simulink model "ACC_Scenario_006_cs"  (R2014b)
settings: Solver=ode5  SolverMode=SingleTasking  StartTime=0.0  StopTime=inf  FixedStep=1/100  RelTol=1e-3
PreLoadFcn:
  | mbxruntime.callbacks.PreLoadFcn(bdroot);
  | check_NUTS_defined;
  | 
  | assignin('base',['model_closed_' bdroot],false);addpath('../includes_ACC');
PostLoadFcn:
  | mbxruntime.callbacks.PostLoadFcn(bdroot);
InitFcn:
  | mbxruntime.callbacks.InitFcn(bdroot);
StartFcn:
  | mbxruntime.callbacks.StartFcn(bdroot);
StopFcn:
  | mbxruntime.callbacks.StopFcn(bdroot);
model workspace: external: MAT-File .\ACC_Scenario_006_cs_hws.mat (data not in the file)
undefined symbols (not defined in the file or in its folder): mbxruntime, OrientationPitch, OrientationRoll, PositionX, PositionY, PositionZ, tabledata, warningInitialVelocity, x0
undefined symbols (not defined in the file): ACC_Scenario_006_cs_061450488d6753c4, ACC_Scenario_006_cs_13896134c615b72a, ACC_Scenario_006_cs_18eaf2a52f2ef75d, ACC_Scenario_006_cs_59e375456829d2f0, ACC_Scenario_006_cs_8a2109b915871f11, ACC_Scenario_006_cs_a4f79cab717c06e2, ACC_Scenario_006_cs_Audi_A8_1_Dynamics_Simple_initialPitch, ACC_Scenario_006_cs_Audi_A8_1_Dynamics_Simple_initialRoll, ACC_Scenario_006_cs_Audi_A8_1_Dynamics_Simple_initialX, ACC_Scenario_006_cs_Audi_A8_1_Dynamics_Simple_initialY, ACC_Scenario_006_cs_Audi_A8_1_Dynamics_Simple_initialYaw, ACC_Scenario_006_cs_Audi_A8_1_Dynamics_Simple_initialZ, ACC_Scenario_006_cs_BMW_X5_1_Path_pathUniqueID, ACC_Scenario_006_cs_BMW_X5_1_SpeedProfile_speedProfileUniqueID, ACC_Scenario_006_cs_e4633c18fd34a832, ACC_Scenario_006_cs_f83c81dc10cd364a, ACC_Scenario_006_cs_Fiat_Bravo_1_Path_pathUniqueID, ACC_Scenario_006_cs_Ford_Fiesta_1_Path_pathUniqueID, ACC_Scenario_006_cs_Honda_Pan_European_1_Path_pathUniqueID, ACC_Scenario_006_cs_Mazda_RX8_1_Path_pathUniqueID, ACC_Scenario_006_cs_Sphere_1_Dynamics_Empty_STATE_Sphere_1_x0, ACC_Scenario_006_cs_Sphere_1_Dynamics_Empty_STATE_Sphere_1_y0, ACC_Scenario_006_cs_Sphere_1_Dynamics_Empty_STATE_Sphere_1_Yaw0, ACC_Scenario_006_cs_Sphere_1_Dynamics_Empty_STATE_Sphere_1_z0, ACC_Scenario_006_cs_Toyota_Yaris_1_Path_pathUniqueID, SteeringColumn, SteeringWheel, Wheel0, Wheel0_Suspension, Wheel1, Wheel1_Suspension, WheelL0, WheelL1, WheelR0, WheelR1
libraries: simulink_extras x60, simulink x21, PreScanSimulinkLibrary x5, PreScanUsefulBlocks x2
(part 6 of 24)

== system ACC_Scenario_006_cs/HighwayOverhang_12 ==
  note: Resources
      |
      | 1: InformationSign\MatrixSign_GreenArrow.png: MatrixSign GreenArrow
      | 2: InformationSign\sign1.jpg: sign1
      | 3: InformationSign\sign2.jpg: sign2
      | 4: InformationSign\sign3.jpg: sign3
      | 5: InformationSign\sign10.png: sign10
      | 7: InformationSign\SEARCH_Logo.png: SEARCH Logo
      | 8: InformationSign\sharp_edges.jpg: sharp edges
      | 9: InformationSign\road_surprises.jpg: road surprises
      | 10: InformationSign\sign5.JPG: sign5
      | 11: InformationSign\tacos.jpg: tacos
      | 12: InformationSign\dont_even_think.jpg: dont even think
      | 13: InformationSign\cthulhuwarn.jpg: cthulhuwarn
      | 14: InformationSign\sign7.JPG: sign7
      | 15: InformationSign\sign32.jpg: sign32
      | 16: InformationSign\NoParking.jpg: NoParking
      | 17: InformationSign\TheFuture.jpg: TheFuture
      | 18: InformationSign\sign4.jpg: sign4
      | 19: InformationSign\sign31.jpg: sign31
      | 20: InformationSign\Empty.jpeg: Empty
  Ground_{1..4} (4 alike) : Ground
  VISUMatrixSignLights_Mux : Subsystem  Tag=mux/VisuMatrixSignLights  mask(PreScan User Interface: VisuMatrixSignLights){}
      mask help:
      | The VisuMatrixSignLights block provides a way to switch the lights on the matrix sign board on or off
      |
      | For more information, please click Help.
      mask Help: eval('openHelp(732)')
  VISUMatrixSign_Mux : Subsystem  Tag=mux/MatrixSign_v2  mask(PreScan User Interface: VisuMatrixSign){}
      mask help:
      | The VisuMatrixSign block provides a way to adapt the texture of the plates connected to an overhang, based on Resource IDs of the texture files.
      |
      | For more information, please click Help.
      settings: DeleteFcn=PreScanBlockDeleteFcn;
      mask Help: eval('openHelp(733)')
  VISUMatrixSign_HighwayOverhang_12 : Outport  Tag=outport/VisuMatrixSign  SampleTime=1/100
  VISUMatrixSignLights_HighwayOverhang_12 : Outport  Tag=outport/VisuMatrixSignLights  Port=2  SampleTime=1/100
  wires:
  VISUMatrixSign_Mux/1(MatrixSigns) -> VISUMatrixSign_HighwayOverhang_12/1
  VISUMatrixSignLights_Mux/1(VISUMatrixSignLights_HighwayOverhang_12) -> VISUMatrixSignLights_HighwayOverhang_12/1
  Ground_1/1 -> VISUMatrixSignLights_Mux/1(MatrixSign_5)
  Ground_2/1 -> VISUMatrixSignLights_Mux/2(MatrixSign_6)
  Ground_3/1 -> VISUMatrixSign_Mux/1(MatrixSign_5)
  Ground_4/1 -> VISUMatrixSign_Mux/2(MatrixSign_6)

== system ACC_Scenario_006_cs/HighwayOverhang_2 ==
  note: Resources
      |
      | 1: InformationSign\MatrixSign_GreenArrow.png: MatrixSign GreenArrow
      | 2: InformationSign\sign1.jpg: sign1
      | 3: InformationSign\sign2.jpg: sign2
      | 4: InformationSign\sign3.jpg: sign3
      | 5: InformationSign\sign10.png: sign10
      | 7: InformationSign\SEARCH_Logo.png: SEARCH Logo
      | 8: InformationSign\sharp_edges.jpg: sharp edges
      | 9: InformationSign\road_surprises.jpg: road surprises
      | 10: InformationSign\sign5.JPG: sign5
      | 11: InformationSign\tacos.jpg: tacos
      | 12: InformationSign\dont_even_think.jpg: dont even think
      | 13: InformationSign\cthulhuwarn.jpg: cthulhuwarn
      | 14: InformationSign\sign7.JPG: sign7
      | 15: InformationSign\sign32.jpg: sign32
      | 16: InformationSign\NoParking.jpg: NoParking
      | 17: InformationSign\TheFuture.jpg: TheFuture
      | 18: InformationSign\sign4.jpg: sign4
      | 19: InformationSign\sign31.jpg: sign31
      | 20: InformationSign\Empty.jpeg: Empty
  Ground_{1..4} (4 alike) : Ground
  VISUMatrixSignLights_Mux : Subsystem  Tag=mux/VisuMatrixSignLights  mask(PreScan User Interface: VisuMatrixSignLights){}
      mask help:
      | The VisuMatrixSignLights block provides a way to switch the lights on the matrix sign board on or off
      |
      | For more information, please click Help.
      mask Help: eval('openHelp(732)')
  VISUMatrixSign_Mux : Subsystem  Tag=mux/MatrixSign_v2  mask(PreScan User Interface: VisuMatrixSign){}
      mask help:
      | The VisuMatrixSign block provides a way to adapt the texture of the plates connected to an overhang, based on Resource IDs of the texture files.
      |
      | For more information, please click Help.
      settings: DeleteFcn=PreScanBlockDeleteFcn;
      mask Help: eval('openHelp(733)')
  VISUMatrixSign_HighwayOverhang_2 : Outport  Tag=outport/VisuMatrixSign  SampleTime=1/100
  VISUMatrixSignLights_HighwayOverhang_2 : Outport  Tag=outport/VisuMatrixSignLights  Port=2  SampleTime=1/100
  wires:
  VISUMatrixSign_Mux/1(MatrixSigns) -> VISUMatrixSign_HighwayOverhang_2/1
  VISUMatrixSignLights_Mux/1(VISUMatrixSignLights_HighwayOverhang_2) -> VISUMatrixSignLights_HighwayOverhang_2/1
  Ground_1/1 -> VISUMatrixSignLights_Mux/1(MatrixSign_3)
  Ground_2/1 -> VISUMatrixSignLights_Mux/2(MatrixSign_4)
  Ground_3/1 -> VISUMatrixSign_Mux/1(MatrixSign_3)
  Ground_4/1 -> VISUMatrixSign_Mux/2(MatrixSign_4)

== system ACC_Scenario_006_cs/HighwayOverhang_3 ==
  note: Resources
      |
      | 1: InformationSign\MatrixSign_GreenArrow.png: MatrixSign GreenArrow
      | 2: InformationSign\sign1.jpg: sign1
      | 3: InformationSign\sign2.jpg: sign2
      | 4: InformationSign\sign3.jpg: sign3
      | 5: InformationSign\sign10.png: sign10
      | 7: InformationSign\SEARCH_Logo.png: SEARCH Logo
      | 8: InformationSign\sharp_edges.jpg: sharp edges
      | 9: InformationSign\road_surprises.jpg: road surprises
      | 10: InformationSign\sign5.JPG: sign5
      | 11: InformationSign\tacos.jpg: tacos
      | 12: InformationSign\dont_even_think.jpg: dont even think
      | 13: InformationSign\cthulhuwarn.jpg: cthulhuwarn
      | 14: InformationSign\sign7.JPG: sign7
      | 15: InformationSign\sign32.jpg: sign32
      | 16: InformationSign\NoParking.jpg: NoParking
      | 17: InformationSign\TheFuture.jpg: TheFuture
      | 18: InformationSign\sign4.jpg: sign4
      | 19: InformationSign\sign31.jpg: sign31
      | 20: InformationSign\Empty.jpeg: Empty
  Ground_1 : Ground
  Ground_2 : Ground
  VISUMatrixSign_Mux : Subsystem  Tag=mux/MatrixSign_v2  mask(PreScan User Interface: VisuMatrixSign){}
      mask help:
      | The VisuMatrixSign block provides a way to adapt the texture of the plates connected to an overhang, based on Resource IDs of the texture files.
      |
      | For more information, please click Help.
      settings: DeleteFcn=PreScanBlockDeleteFcn;
      mask Help: eval('openHelp(733)')
  VISUMatrixSign_HighwayOverhang_3 : Outport  Tag=outport/VisuMatrixSign  SampleTime=1/100
  wires:
  VISUMatrixSign_Mux/1(MatrixSigns) -> VISUMatrixSign_HighwayOverhang_3/1
  Ground_1/1 -> VISUMatrixSign_Mux/1(InformationPlate_1)
  Ground_2/1 -> VISUMatrixSign_Mux/2(InformationPlate_2)

== system ACC_Scenario_006_cs/HighwayOverhang_4 ==
  note: Resources
      |
      | 1: InformationSign\MatrixSign_GreenArrow.png: MatrixSign GreenArrow
      | 2: InformationSign\sign1.jpg: sign1
      | 3: InformationSign\sign2.jpg: sign2
      | 4: InformationSign\sign3.jpg: sign3
      | 5: InformationSign\sign10.png: sign10
      | 7: InformationSign\SEARCH_Logo.png: SEARCH Logo
      | 8: InformationSign\sharp_edges.jpg: sharp edges
      | 9: InformationSign\road_surprises.jpg: road surprises
      | 10: InformationSign\sign5.JPG: sign5
      | 11: InformationSign\tacos.jpg: tacos
      | 12: InformationSign\dont_even_think.jpg: dont even think
      | 13: InformationSign\cthulhuwarn.jpg: cthulhuwarn
      | 14: InformationSign\sign7.JPG: sign7
      | 15: InformationSign\sign32.jpg: sign32
      | 16: InformationSign\NoParking.jpg: NoParking
      | 17: InformationSign\TheFuture.jpg: TheFuture
      | 18: InformationSign\sign4.jpg: sign4
      | 19: InformationSign\sign31.jpg: sign31
      | 20: InformationSign\Empty.jpeg: Empty
  Ground_1 : Ground
  Ground_2 : Ground
  VISUMatrixSign_Mux : Subsystem  Tag=mux/MatrixSign_v2  mask(PreScan User Interface: VisuMatrixSign){}
      mask help:
      | The VisuMatrixSign block provides a way to adapt the texture of the plates connected to an overhang, based on Resource IDs of the texture files.
      |
      | For more information, please click Help.
      settings: DeleteFcn=PreScanBlockDeleteFcn;
      mask Help: eval('openHelp(733)')
  VISUMatrixSign_HighwayOverhang_4 : Outport  Tag=outport/VisuMatrixSign  SampleTime=1/100
  wires:
  VISUMatrixSign_Mux/1(MatrixSigns) -> VISUMatrixSign_HighwayOverhang_4/1
  Ground_1/1 -> VISUMatrixSign_Mux/1(InformationPlate_3)
  Ground_2/1 -> VISUMatrixSign_Mux/2(InformationPlate_4)

== system ACC_Scenario_006_cs/HighwayOverhang_5 ==
  note: Resources
      |
      | 1: InformationSign\MatrixSign_GreenArrow.png: MatrixSign GreenArrow
      | 2: InformationSign\sign1.jpg: sign1
      | 3: InformationSign\sign2.jpg: sign2
      | 4: InformationSign\sign3.jpg: sign3
      | 5: InformationSign\sign10.png: sign10
      | 7: InformationSign\SEARCH_Logo.png: SEARCH Logo
      | 8: InformationSign\sharp_edges.jpg: sharp edges
      | 9: InformationSign\road_surprises.jpg: road surprises
      | 10: InformationSign\sign5.JPG: sign5
      | 11: InformationSign\tacos.jpg: tacos
      | 12: InformationSign\dont_even_think.jpg: dont even think
      | 13: InformationSign\cthulhuwarn.jpg: cthulhuwarn
      | 14: InformationSign\sign7.JPG: sign7
      | 15: InformationSign\sign32.jpg: sign32
      | 16: InformationSign\NoParking.jpg: NoParking
      | 17: InformationSign\TheFuture.jpg: TheFuture
      | 18: InformationSign\sign4.jpg: sign4
      | 19: InformationSign\sign31.jpg: sign31
      | 20: InformationSign\Empty.jpeg: Empty
  Ground_1 : Ground
  Ground_2 : Ground
  VISUMatrixSign_Mux : Subsystem  Tag=mux/MatrixSign_v2  mask(PreScan User Interface: VisuMatrixSign){}
      mask help:
      | The VisuMatrixSign block provides a way to adapt the texture of the plates connected to an overhang, based on Resource IDs of the texture files.
      |
      | For more information, please click Help.
      settings: DeleteFcn=PreScanBlockDeleteFcn;
      mask Help: eval('openHelp(733)')
  VISUMatrixSign_HighwayOverhang_5 : Outport  Tag=outport/VisuMatrixSign  SampleTime=1/100
  wires:
  VISUMatrixSign_Mux/1(MatrixSigns) -> VISUMatrixSign_HighwayOverhang_5/1
  Ground_1/1 -> VISUMatrixSign_Mux/1(InformationPlate_5)
  Ground_2/1 -> VISUMatrixSign_Mux/2(InformationPlate_6)

== system ACC_Scenario_006_cs/HighwayOverhang_6 ==
  note: Resources
      |
      | 1: InformationSign\MatrixSign_GreenArrow.png: MatrixSign GreenArrow
      | 2: InformationSign\sign1.jpg: sign1
      | 3: InformationSign\sign2.jpg: sign2
      | 4: InformationSign\sign3.jpg: sign3
      | 5: InformationSign\sign10.png: sign10
      | 7: InformationSign\SEARCH_Logo.png: SEARCH Logo
      | 8: InformationSign\sharp_edges.jpg: sharp edges
      | 9: InformationSign\road_surprises.jpg: road surprises
      | 10: InformationSign\sign5.JPG: sign5
      | 11: InformationSign\tacos.jpg: tacos
      | 12: InformationSign\dont_even_think.jpg: dont even think
      | 13: InformationSign\cthulhuwarn.jpg: cthulhuwarn
      | 14: InformationSign\sign7.JPG: sign7
      | 15: InformationSign\sign32.jpg: sign32
      | 16: InformationSign\NoParking.jpg: NoParking
      | 17: InformationSign\TheFuture.jpg: TheFuture
      | 18: InformationSign\sign4.jpg: sign4
      | 19: InformationSign\sign31.jpg: sign31
      | 20: InformationSign\Empty.jpeg: Empty
  Ground_1 : Ground
  Ground_2 : Ground
  VISUMatrixSign_Mux : Subsystem  Tag=mux/MatrixSign_v2  mask(PreScan User Interface: VisuMatrixSign){}
      mask help:
      | The VisuMatrixSign block provides a way to adapt the texture of the plates connected to an overhang, based on Resource IDs of the texture files.
      |
      | For more information, please click Help.
      settings: DeleteFcn=PreScanBlockDeleteFcn;
      mask Help: eval('openHelp(733)')
  VISUMatrixSign_HighwayOverhang_6 : Outport  Tag=outport/VisuMatrixSign  SampleTime=1/100
  wires:
  VISUMatrixSign_Mux/1(MatrixSigns) -> VISUMatrixSign_HighwayOverhang_6/1
  Ground_1/1 -> VISUMatrixSign_Mux/1(InformationPlate_7)
  Ground_2/1 -> VISUMatrixSign_Mux/2(InformationPlate_8)

== system ACC_Scenario_006_cs/HighwayOverhang_7 ==
  note: Resources
      |
      | 1: InformationSign\MatrixSign_GreenArrow.png: MatrixSign GreenArrow
      | 2: InformationSign\sign1.jpg: sign1
      | 3: InformationSign\sign2.jpg: sign2
      | 4: InformationSign\sign3.jpg: sign3
      | 5: InformationSign\sign10.png: sign10
      | 7: InformationSign\SEARCH_Logo.png: SEARCH Logo
      | 8: InformationSign\sharp_edges.jpg: sharp edges
      | 9: InformationSign\road_surprises.jpg: road surprises
      | 10: InformationSign\sign5.JPG: sign5
      | 11: InformationSign\tacos.jpg: tacos
      | 12: InformationSign\dont_even_think.jpg: dont even think
      | 13: InformationSign\cthulhuwarn.jpg: cthulhuwarn
      | 14: InformationSign\sign7.JPG: sign7
      | 15: InformationSign\sign32.jpg: sign32
      | 16: InformationSign\NoParking.jpg: NoParking
      | 17: InformationSign\TheFuture.jpg: TheFuture
      | 18: InformationSign\sign4.jpg: sign4
      | 19: InformationSign\sign31.jpg: sign31
      | 20: InformationSign\Empty.jpeg: Empty
  Ground_1 : Ground
  Ground_2 : Ground
  VISUMatrixSign_Mux : Subsystem  Tag=mux/MatrixSign_v2  mask(PreScan User Interface: VisuMatrixSign){}
      mask help:
      | The VisuMatrixSign block provides a way to adapt the texture of the plates connected to an overhang, based on Resource IDs of the texture files.
      |
      | For more information, please click Help.
      settings: DeleteFcn=PreScanBlockDeleteFcn;
      mask Help: eval('openHelp(733)')
  VISUMatrixSign_HighwayOverhang_7 : Outport  Tag=outport/VisuMatrixSign  SampleTime=1/100
  wires:
  VISUMatrixSign_Mux/1(MatrixSigns) -> VISUMatrixSign_HighwayOverhang_7/1
  Ground_1/1 -> VISUMatrixSign_Mux/1(InformationPlate_9)
  Ground_2/1 -> VISUMatrixSign_Mux/2(InformationPlate_10)

== system ACC_Scenario_006_cs/HighwayOverhang_8 ==
  note: Resources
      |
      | 1: InformationSign\MatrixSign_GreenArrow.png: MatrixSign GreenArrow
      | 2: InformationSign\sign1.jpg: sign1
      | 3: InformationSign\sign2.jpg: sign2
      | 4: InformationSign\sign3.jpg: sign3
      | 5: InformationSign\sign10.png: sign10
      | 7: InformationSign\SEARCH_Logo.png: SEARCH Logo
      | 8: InformationSign\sharp_edges.jpg: sharp edges
      | 9: InformationSign\road_surprises.jpg: road surprises
      | 10: InformationSign\sign5.JPG: sign5
      | 11: InformationSign\tacos.jpg: tacos
      | 12: InformationSign\dont_even_think.jpg: dont even think
      | 13: InformationSign\cthulhuwarn.jpg: cthulhuwarn
      | 14: InformationSign\sign7.JPG: sign7
      | 15: InformationSign\sign32.jpg: sign32
      | 16: InformationSign\NoParking.jpg: NoParking
      | 17: InformationSign\TheFuture.jpg: TheFuture
      | 18: InformationSign\sign4.jpg: sign4
      | 19: InformationSign\sign31.jpg: sign31
      | 20: InformationSign\Empty.jpeg: Empty
  Ground_1 : Ground
  Ground_2 : Ground
  VISUMatrixSign_Mux : Subsystem  Tag=mux/MatrixSign_v2  mask(PreScan User Interface: VisuMatrixSign){}
      mask help:
      | The VisuMatrixSign block provides a way to adapt the texture of the plates connected to an overhang, based on Resource IDs of the texture files.
      |
      | For more information, please click Help.
      settings: DeleteFcn=PreScanBlockDeleteFcn;
      mask Help: eval('openHelp(733)')
  VISUMatrixSign_HighwayOverhang_8 : Outport  Tag=outport/VisuMatrixSign  SampleTime=1/100
  wires:
  VISUMatrixSign_Mux/1(MatrixSigns) -> VISUMatrixSign_HighwayOverhang_8/1
  Ground_1/1 -> VISUMatrixSign_Mux/1(InformationPlate_11)
  Ground_2/1 -> VISUMatrixSign_Mux/2(InformationPlate_12)

== system ACC_Scenario_006_cs/HighwayOverhang_9 ==
  note: Resources
      |
      | 1: InformationSign\MatrixSign_GreenArrow.png: MatrixSign GreenArrow
      | 2: InformationSign\sign1.jpg: sign1
      | 3: InformationSign\sign2.jpg: sign2
      | 4: InformationSign\sign3.jpg: sign3
      | 5: InformationSign\sign10.png: sign10
      | 7: InformationSign\SEARCH_Logo.png: SEARCH Logo
      | 8: InformationSign\sharp_edges.jpg: sharp edges
      | 9: InformationSign\road_surprises.jpg: road surprises
      | 10: InformationSign\sign5.JPG: sign5
      | 11: InformationSign\tacos.jpg: tacos
      | 12: InformationSign\dont_even_think.jpg: dont even think
      | 13: InformationSign\cthulhuwarn.jpg: cthulhuwarn
      | 14: InformationSign\sign7.JPG: sign7
      | 15: InformationSign\sign32.jpg: sign32
      | 16: InformationSign\NoParking.jpg: NoParking
      | 17: InformationSign\TheFuture.jpg: TheFuture
      | 18: InformationSign\sign4.jpg: sign4
      | 19: InformationSign\sign31.jpg: sign31
      | 20: InformationSign\Empty.jpeg: Empty
  Ground_1 : Ground
  Ground_2 : Ground
  VISUMatrixSign_Mux : Subsystem  Tag=mux/MatrixSign_v2  mask(PreScan User Interface: VisuMatrixSign){}
      mask help:
      | The VisuMatrixSign block provides a way to adapt the texture of the plates connected to an overhang, based on Resource IDs of the texture files.
      |
      | For more information, please click Help.
      settings: DeleteFcn=PreScanBlockDeleteFcn;
      mask Help: eval('openHelp(733)')
  VISUMatrixSign_HighwayOverhang_9 : Outport  Tag=outport/VisuMatrixSign  SampleTime=1/100
  wires:
  VISUMatrixSign_Mux/1(MatrixSigns) -> VISUMatrixSign_HighwayOverhang_9/1
  Ground_1/1 -> VISUMatrixSign_Mux/1(InformationPlate_13)
  Ground_2/1 -> VISUMatrixSign_Mux/2(InformationPlate_14)

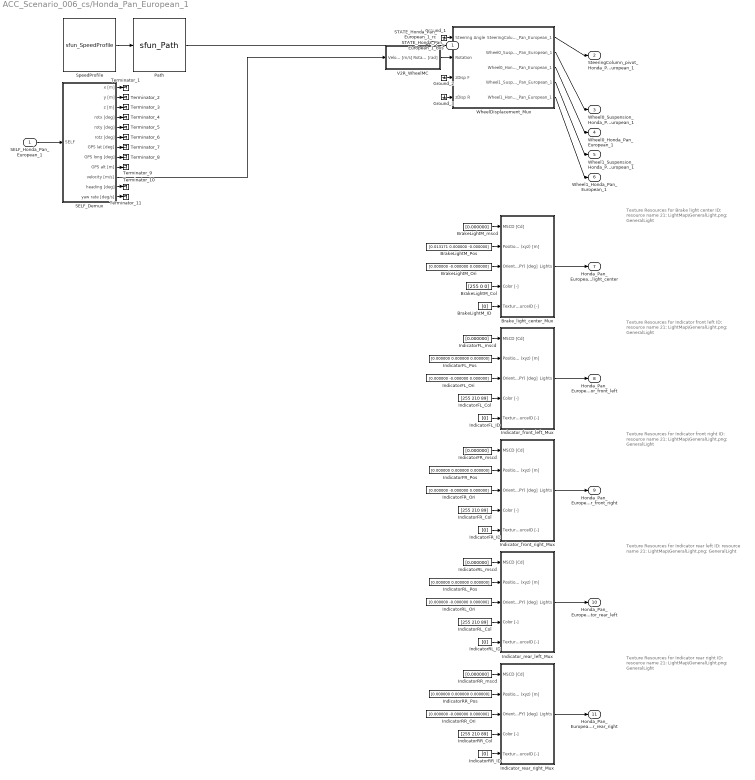
== system ACC_Scenario_006_cs/Honda_Pan_European_1 ==
  note: Texture Resources for Brake light center
      |
      | ID: resource name
      | 21: LightMap\GeneralLight.png: GeneralLight
  note: Texture Resources for Indicator front left
      |
      | ID: resource name
      | 21: LightMap\GeneralLight.png: GeneralLight
  note: Texture Resources for Indicator front right
      |
      | ID: resource name
      | 21: LightMap\GeneralLight.png: GeneralLight
  note: Texture Resources for Indicator rear left
      |
      | ID: resource name
      | 21: LightMap\GeneralLight.png: GeneralLight
  note: Texture Resources for Indicator rear right
      |
      | ID: resource name
      | 21: LightMap\GeneralLight.png: GeneralLight
  SELF_Honda_Pan_European_1 : Inport  Tag=inport/SelfPort  OutDataTypeStr=Bus: PRESCAN_SELFSENSORDATA  PortDimensions=1  SampleTime=1/100  BusOutputAsStruct=on
  BrakeLightM_Col : Constant  Tag=VisuLightConst  Value=[255 0 0]
  BrakeLightM_ID : Constant  Tag=VisuLightConst  Value=[0]
  BrakeLightM_Ori : Constant  Tag=VisuLightConst  Value=[0.000000 -0.000000 0.000000]
  BrakeLightM_Pos : Constant  Tag=VisuLightConst  Value=[0.013171 0.000000 -0.000000]
  BrakeLightM_mscd : Constant  Tag=VisuLightConst  Value=[0.000000]
  Brake_light_center_Mux : Subsystem  Tag=mux/ActiveLight  mask(PreScan User Interface: VisuActiveLight){}
      mask help:
      | The VisuActiveLight block provides a way for detailed animation of Light Sources, such as the indicator, brake, fog and main lights of a vehicle, or a light post.
      |
      | For more information, please click Help.
      settings: DeleteFcn=PreScanBlockDeleteFcn;
      mask Help: eval('openHelp(209)')
  Ground_1 : Ground
  Ground_2 : Ground
  Ground_3 : Ground
  IndicatorFL_Col : Constant  Tag=VisuLightConst  Value=[255 210 89]
  IndicatorFL_ID : Constant  Tag=VisuLightConst  Value=[0]
  IndicatorFL_Ori : Constant  Tag=VisuLightConst  Value=[0.000000 -0.000000 0.000000]
  IndicatorFL_Pos : Constant  Tag=VisuLightConst  Value=[0.000000 0.000000 0.000000]
  IndicatorFL_mscd : Constant  Tag=VisuLightConst  Value=[0.000000]
  IndicatorFR_Col : Constant  Tag=VisuLightConst  Value=[255 210 89]
  IndicatorFR_ID : Constant  Tag=VisuLightConst  Value=[0]
  IndicatorFR_Ori : Constant  Tag=VisuLightConst  Value=[0.000000 -0.000000 0.000000]
  IndicatorFR_Pos : Constant  Tag=VisuLightConst  Value=[0.000000 0.000000 0.000000]
  IndicatorFR_mscd : Constant  Tag=VisuLightConst  Value=[0.000000]
  IndicatorRL_Col : Constant  Tag=VisuLightConst  Value=[255 210 89]
  IndicatorRL_ID : Constant  Tag=VisuLightConst  Value=[0]
  IndicatorRL_Ori : Constant  Tag=VisuLightConst  Value=[0.000000 -0.000000 0.000000]
  IndicatorRL_Pos : Constant  Tag=VisuLightConst  Value=[0.000000 0.000000 0.000000]
  IndicatorRL_mscd : Constant  Tag=VisuLightConst  Value=[0.000000]
  IndicatorRR_Col : Constant  Tag=VisuLightConst  Value=[255 210 89]
  IndicatorRR_ID : Constant  Tag=VisuLightConst  Value=[0]
  IndicatorRR_Ori : Constant  Tag=VisuLightConst  Value=[0.000000 -0.000000 0.000000]
  IndicatorRR_Pos : Constant  Tag=VisuLightConst  Value=[0.000000 0.000000 0.000000]
  IndicatorRR_mscd : Constant  Tag=VisuLightConst  Value=[0.000000]
  Indicator_front_left_Mux : Subsystem  Tag=mux/ActiveLight  mask(PreScan User Interface: VisuActiveLight){}
      mask help:
      | The VisuActiveLight block provides a way for detailed animation of Light Sources, such as the indicator, brake, fog and main lights of a vehicle, or a light post.
      |
      | For more information, please click Help.
      settings: DeleteFcn=PreScanBlockDeleteFcn;
      mask Help: eval('openHelp(209)')
  Indicator_front_right_Mux : Subsystem  Tag=mux/ActiveLight  mask(PreScan User Interface: VisuActiveLight){}
      mask help:
      | The VisuActiveLight block provides a way for detailed animation of Light Sources, such as the indicator, brake, fog and main lights of a vehicle, or a light post.
      |
      | For more information, please click Help.
      settings: DeleteFcn=PreScanBlockDeleteFcn;
      mask Help: eval('openHelp(209)')
  Indicator_rear_left_Mux : Subsystem  Tag=mux/ActiveLight  mask(PreScan User Interface: VisuActiveLight){}
      mask help:
      | The VisuActiveLight block provides a way for detailed animation of Light Sources, such as the indicator, brake, fog and main lights of a vehicle, or a light post.
      |
      | For more information, please click Help.
      settings: DeleteFcn=PreScanBlockDeleteFcn;
      mask Help: eval('openHelp(209)')
  Indicator_rear_right_Mux : Subsystem  Tag=mux/ActiveLight  mask(PreScan User Interface: VisuActiveLight){}
      mask help:
      | The VisuActiveLight block provides a way for detailed animation of Light Sources, such as the indicator, brake, fog and main lights of a vehicle, or a light post.
      |
      | For more information, please click Help.
      settings: DeleteFcn=PreScanBlockDeleteFcn;
      mask Help: eval('openHelp(209)')
  Path : S-Function  Tag=Path  LoadFcn=load('PrescanMotionData.mat')  FunctionName=sfun_Path  Parameters=uniqueID, pathUniqueID, timestep  EnableBusSupport=off  mask(Path){uniqueID=356, pathUniqueID=ACC_Scenario_006_cs_Honda_Pan_European_1_Path_pathUniqueID, timestep=1/100}
      mask prompts: uniqueID "Object Unique ID"; pathUniqueID "Path Unique ID"; timestep "MATLAB timestep:"
      mask help:
      | The path block outputs the position along a given trajectory.
      |
      | For more information, please click Help.
      mask Help: eval('openHelp(312)')
      mask Display: image(imread('Path.png'))
  SELF_Demux : Subsystem  Tag=demux/SelfPort  mask(PreScan Demux Block:){}
      mask help:
      | The SELF port shows (state) information of the actor itself. The outputs are position in the experiment's axis system and the GPS coordinates, and the object's absolute velocity and compass heading.
      |
      | For more information, please click Help.
      settings: DeleteFcn=PreScanBlockDeleteFcn;
      mask Help: eval('openHelp(462)')
      mask Display:
      | port_label('output',1,'x [m]')
      | port_label('output',2,'y [m]')
      | port_label('output',3,'z [m]','texmode','on')
      | port_label('output',4,'Rotx [deg]','texmode','on')
      | port_label('output',5,'Roty [deg]','texmode','on')
      | port_label('output',6,'Rotz [deg]','texmode','on')
      | port_label('output',7,'GPS lat [deg]','texmode','on')
      | port_label('output',8,'GPS long [deg]','texmode','on')
      | port_label('output',9,'GPS alt [m]','texmode','on')
      | port_label('output',10,'Velocity [m/s]')
      | port_label('output',11,'Heading [deg]')
      | port_label('output',12,'Yaw rate [deg/s]')
  STATE_Honda_Pan_European_1_rc : RateTransition  Tag=mux_rc/StatePort  OutPortSampleTimeOpt=Inherit
  SpeedProfile : S-Function  Tag=SpeedProfile  LoadFcn=load('PrescanMotionData.mat')  FunctionName=sfun_SpeedProfile  Parameters=speedProfileUniqueID, timestep  EnableBusSupport=off  mask(SpeedProfile){speedProfileUniqueID=ACC_Scenario_006_cs_59e375456829d2f0, timestep=1/100}
      mask prompts: speedProfileUniqueID "Speed Profile Unique ID"; timestep "MATLAB timestep:"
      mask help:
      | The speed profile block outputs the travelled distance, velocities and acceleration along a given path.
      |
      | For more information, please click Help.
      mask Help: eval('openHelp(312)')
      mask Display: image(imread('SpeedProfile.png'))
  Terminator_{1..11} (11 alike) : Terminator
  V2R_WheelMC : Subsystem  Tag=mux/Wheels  mask(PreScan Velocity to Wheel Angle Block:){TimeStep=-1, TireRadius=0.29}
      mask prompts: TimeStep "Auto Assigned: Time Step [s]"; TireRadius "Tire Radius [m]"
      settings: DeleteFcn=PreScanBlockDeleteFcn;
      mask Display: disp('Velocity\nto\nWheelAngle')
  WheelDisplacement_Mux : Subsystem  Tag=mux/JointGroup  mask(JointGroup){}
      mask help:
      | The JointGroup allows to control several Joints in one go, as defined for this particular model.
      | For more information, look in the PreScan manual in the section "Model Preparation Tool" -> "Joint Groups"
      |
      | For more information on the Joints simulink interface, press Help.
      mask Help: eval('openHelp(254)')
  STATE_Honda_Pan_European_1_bus : Outport  Tag=outport/StatePort  OutDataTypeStr=Bus: PRESCAN_STATEACTUATORDATA  PortDimensions=1  SampleTime=1/100
  SteeringColumn_pivot_Honda_Pan_European_1 : Outport  Tag=outport/JointActuator  Port=2  OutDataTypeStr=Bus: PRESCAN_POSE_DATA  SampleTime=1/100
  Wheel0_Suspension_Honda_Pan_European_1 : Outport  Tag=outport/JointActuator  Port=3  OutDataTypeStr=Bus: PRESCAN_POSE_DATA  SampleTime=1/100
  Wheel0_Honda_Pan_European_1 : Outport  Tag=outport/JointActuator  Port=4  OutDataTypeStr=Bus: PRESCAN_POSE_DATA  SampleTime=1/100
  Wheel1_Suspension_Honda_Pan_European_1 : Outport  Tag=outport/JointActuator  Port=5  OutDataTypeStr=Bus: PRESCAN_POSE_DATA  SampleTime=1/100
  Wheel1_Honda_Pan_European_1 : Outport  Tag=outport/JointActuator  Port=6  OutDataTypeStr=Bus: PRESCAN_POSE_DATA  SampleTime=1/100
  Honda_Pan_European_1_Brake_light_center : Outport  Tag=outport/BrakeLightM  Port=7  OutDataTypeStr=Bus: PRESCAN_VISULIGHTACTUATOR_DATA  SampleTime=1/100
  Honda_Pan_European_1_Indicator_front_left : Outport  Tag=outport/IndicatorFL  Port=8  OutDataTypeStr=Bus: PRESCAN_VISULIGHTACTUATOR_DATA  SampleTime=1/100
  Honda_Pan_European_1_Indicator_front_right : Outport  Tag=outport/IndicatorFR  Port=9  OutDataTypeStr=Bus: PRESCAN_VISULIGHTACTUATOR_DATA  SampleTime=1/100
  Honda_Pan_European_1_Indicator_rear_left : Outport  Tag=outport/IndicatorRL  Port=10  OutDataTypeStr=Bus: PRESCAN_VISULIGHTACTUATOR_DATA  SampleTime=1/100
  Honda_Pan_European_1_Indicator_rear_right : Outport  Tag=outport/IndicatorRR  Port=11  OutDataTypeStr=Bus: PRESCAN_VISULIGHTACTUATOR_DATA  SampleTime=1/100
  wires:
  V2R_WheelMC/1(Rotation [rad]) -> WheelDisplacement_Mux/2(Rotation)
  SELF_Demux/10(velocity [m/s]) -> V2R_WheelMC/1(Velocity [m/s])
  STATE_Honda_Pan_European_1_rc/1 -> STATE_Honda_Pan_European_1_bus/1
  SpeedProfile/1 -> Path/1
  Path/1 -> STATE_Honda_Pan_European_1_rc/1
  SELF_Honda_Pan_European_1/1 -> SELF_Demux/1(SELF)
  WheelDisplacement_Mux/1(SteeringColumn_pivot_Honda_Pan_European_1) -> SteeringColumn_pivot_Honda_Pan_European_1/1
  WheelDisplacement_Mux/2(Wheel0_Suspension_Honda_Pan_European_1) -> Wheel0_Suspension_Honda_Pan_European_1/1
  WheelDisplacement_Mux/3(Wheel0_Honda_Pan_European_1) -> Wheel0_Honda_Pan_European_1/1
  WheelDisplacement_Mux/4(Wheel1_Suspension_Honda_Pan_European_1) -> Wheel1_Suspension_Honda_Pan_European_1/1
  WheelDisplacement_Mux/5(Wheel1_Honda_Pan_European_1) -> Wheel1_Honda_Pan_European_1/1
  Brake_light_center_Mux/1(Lights) -> Honda_Pan_European_1_Brake_light_center/1
  BrakeLightM_mscd/1 -> Brake_light_center_Mux/1(MSCD [Cd])
  BrakeLightM_Pos/1 -> Brake_light_center_Mux/2(Position (xyz) [m])
  BrakeLightM_Ori/1 -> Brake_light_center_Mux/3(Orientation (RPY) [deg])
  BrakeLightM_Col/1 -> Brake_light_center_Mux/4(Color [-])
  BrakeLightM_ID/1 -> Brake_light_center_Mux/5(TextureResourceID [-])
  Indicator_front_left_Mux/1(Lights) -> Honda_Pan_European_1_Indicator_front_left/1
  IndicatorFL_mscd/1 -> Indicator_front_left_Mux/1(MSCD [Cd])
  IndicatorFL_Pos/1 -> Indicator_front_left_Mux/2(Position (xyz) [m])
  IndicatorFL_Ori/1 -> Indicator_front_left_Mux/3(Orientation (RPY) [deg])
  IndicatorFL_Col/1 -> Indicator_front_left_Mux/4(Color [-])
  IndicatorFL_ID/1 -> Indicator_front_left_Mux/5(TextureResourceID [-])
  Indicator_front_right_Mux/1(Lights) -> Honda_Pan_European_1_Indicator_front_right/1
  IndicatorFR_mscd/1 -> Indicator_front_right_Mux/1(MSCD [Cd])
  IndicatorFR_Pos/1 -> Indicator_front_right_Mux/2(Position (xyz) [m])
  IndicatorFR_Ori/1 -> Indicator_front_right_Mux/3(Orientation (RPY) [deg])
  IndicatorFR_Col/1 -> Indicator_front_right_Mux/4(Color [-])
  IndicatorFR_ID/1 -> Indicator_front_right_Mux/5(TextureResourceID [-])
  Indicator_rear_left_Mux/1(Lights) -> Honda_Pan_European_1_Indicator_rear_left/1
  IndicatorRL_mscd/1 -> Indicator_rear_left_Mux/1(MSCD [Cd])
  IndicatorRL_Pos/1 -> Indicator_rear_left_Mux/2(Position (xyz) [m])
  IndicatorRL_Ori/1 -> Indicator_rear_left_Mux/3(Orientation (RPY) [deg])
  IndicatorRL_Col/1 -> Indicator_rear_left_Mux/4(Color [-])
  IndicatorRL_ID/1 -> Indicator_rear_left_Mux/5(TextureResourceID [-])
  Indicator_rear_right_Mux/1(Lights) -> Honda_Pan_European_1_Indicator_rear_right/1
  IndicatorRR_mscd/1 -> Indicator_rear_right_Mux/1(MSCD [Cd])
  IndicatorRR_Pos/1 -> Indicator_rear_right_Mux/2(Position (xyz) [m])
  IndicatorRR_Ori/1 -> Indicator_rear_right_Mux/3(Orientation (RPY) [deg])
  IndicatorRR_Col/1 -> Indicator_rear_right_Mux/4(Color [-])
  IndicatorRR_ID/1 -> Indicator_rear_right_Mux/5(TextureResourceID [-])
  SELF_Demux/1(x [m]) -> Terminator_1/1
  SELF_Demux/2(y [m]) -> Terminator_2/1
  SELF_Demux/3(z [m]) -> Terminator_3/1
  SELF_Demux/4(rotx [deg]) -> Terminator_4/1
  SELF_Demux/5(roty [deg]) -> Terminator_5/1
  SELF_Demux/6(rotz [deg]) -> Terminator_6/1
  SELF_Demux/7(GPS lat [deg]) -> Terminator_7/1
  SELF_Demux/8(GPS long [deg]) -> Terminator_8/1
  SELF_Demux/9(GPS alt [m]) -> Terminator_9/1
  SELF_Demux/11(heading [deg]) -> Terminator_10/1
  SELF_Demux/12(yaw rate [deg/s]) -> Terminator_11/1
  Ground_1/1 -> WheelDisplacement_Mux/1(Steering Angle)
  Ground_2/1 -> WheelDisplacement_Mux/3(zDisp F)
  Ground_3/1 -> WheelDisplacement_Mux/4(zDisp R)

== system ACC_Scenario_006_cs/Honda_Pan_European_1_Brake_light_center ==
  Honda_Pan_European_1_Brake_light_center : Inport  Tag=inport/BrakeLightM  OutDataTypeStr=Bus: PRESCAN_VISULIGHTACTUATOR_DATA  SampleTime=1/100  BusOutputAsStruct=on
  Actuator : S-Function  FunctionName=sfun_VisuLightActuator  Parameters=mbxruntime.parameters.convert(UniqueID), mbxruntime.parameters.convert(LightName), mbxruntime.parameters.convert(PivotName), mbxruntime.parameters.convert(TextureResources), mbxruntime.parameters.convert(ColorsObjectName), mbxruntime.parameters.convert(MeshOnColor), mbxruntime.parameters.convert(MeshOffColor),tabledata, TimeStep  EnableBusSupport=off  mask(PreScan Sink Block: VisuActiveLight){UniqueID=356, LightName=Honda_Pan_European_1.LightActuator_0_BrakeLightM_ActiveLight, PivotName=Honda_Pan_European_1.BrakeLightM_pivot, TextureResources={ '21' 'LightMap\GeneralLight.png'}, ColorsObjectName=Honda_Pan_European_1.BrakeLightM, MeshOnColor=[255    0    0  255  255    0    0  255  102  102  102  255  510    0    0  255], MeshOffColor=[255    0    0  255  255    0    0  255  102  102  102  255    0    0    0  255], TimeStep=1/100}
      mask prompts: UniqueID "Parent Unique Identifier"; LightName "Light"; PivotName "Pivot"; TextureResources "Texture Resources"; ColorsObjectName "Light Fixture Color Object"; MeshOnColor "Light Fixture On Color"; MeshOffColor "Light Fixture Off Color"; TimeStep "Simulink time step"
      mask help:
      | The VisuActiveLight block provides a way for detailed animation of Light Sources, such as the indicator, brake, fog and main lights of a vehicle, or a light post.
      |
      | For more information, please click Help.
      mask init:
      | [tabledata] = mbxruntime.parameters.table(UniqueID,LightName,PivotName,TextureResources,ColorsObjectName,MeshOnColor,MeshOffColor);
      mask Help: eval('openHelp(209)')
      mask Display: image(imread('HeadLight.png'))
  wires:
  Honda_Pan_European_1_Brake_light_center/1 -> Actuator/1

== system ACC_Scenario_006_cs/Honda_Pan_European_1_Indicator_front_left ==
  Honda_Pan_European_1_Indicator_front_left : Inport  Tag=inport/IndicatorFL  OutDataTypeStr=Bus: PRESCAN_VISULIGHTACTUATOR_DATA  SampleTime=1/100  BusOutputAsStruct=on
  Actuator : S-Function  FunctionName=sfun_VisuLightActuator  Parameters=mbxruntime.parameters.convert(UniqueID), mbxruntime.parameters.convert(LightName), mbxruntime.parameters.convert(PivotName), mbxruntime.parameters.convert(TextureResources), mbxruntime.parameters.convert(ColorsObjectName), mbxruntime.parameters.convert(MeshOnColor), mbxruntime.parameters.convert(MeshOffColor),tabledata, TimeStep  EnableBusSupport=off  mask(PreScan Sink Block: VisuActiveLight){UniqueID=356, LightName=Honda_Pan_European_1.LightActuator_1_IndicatorFL_ActiveLight, PivotName=Honda_Pan_European_1.IndicatorFL_pivot, TextureResources={ '21' 'LightMap\GeneralLight.png'}, ColorsObjectName=Honda_Pan_European_1.IndicatorFL, MeshOnColor=[255  165    0    0  255  165    0    0  102  102  102  255  510  420  178  255], MeshOffColor=[255  165    0    0  255  165    0    0  102  102  102  255    0    0    0  255], TimeStep=1/100}
      mask prompts: UniqueID "Parent Unique Identifier"; LightName "Light"; PivotName "Pivot"; TextureResources "Texture Resources"; ColorsObjectName "Light Fixture Color Object"; MeshOnColor "Light Fixture On Color"; MeshOffColor "Light Fixture Off Color"; TimeStep "Simulink time step"
      mask help:
      | The VisuActiveLight block provides a way for detailed animation of Light Sources, such as the indicator, brake, fog and main lights of a vehicle, or a light post.
      |
      | For more information, please click Help.
      mask init:
      | [tabledata] = mbxruntime.parameters.table(UniqueID,LightName,PivotName,TextureResources,ColorsObjectName,MeshOnColor,MeshOffColor);
      mask Help: eval('openHelp(209)')
      mask Display: image(imread('HeadLight.png'))
  wires:
  Honda_Pan_European_1_Indicator_front_left/1 -> Actuator/1

== system ACC_Scenario_006_cs/Honda_Pan_European_1_Indicator_front_right ==
  Honda_Pan_European_1_Indicator_front_right : Inport  Tag=inport/IndicatorFR  OutDataTypeStr=Bus: PRESCAN_VISULIGHTACTUATOR_DATA  SampleTime=1/100  BusOutputAsStruct=on
  Actuator : S-Function  FunctionName=sfun_VisuLightActuator  Parameters=mbxruntime.parameters.convert(UniqueID), mbxruntime.parameters.convert(LightName), mbxruntime.parameters.convert(PivotName), mbxruntime.parameters.convert(TextureResources), mbxruntime.parameters.convert(ColorsObjectName), mbxruntime.parameters.convert(MeshOnColor), mbxruntime.parameters.convert(MeshOffColor),tabledata, TimeStep  EnableBusSupport=off  mask(PreScan Sink Block: VisuActiveLight){UniqueID=356, LightName=Honda_Pan_European_1.LightActuator_2_IndicatorFR_ActiveLight, PivotName=Honda_Pan_European_1.IndicatorFR_pivot, TextureResources={ '21' 'LightMap\GeneralLight.png'}, ColorsObjectName=Honda_Pan_European_1.IndicatorFR, MeshOnColor=[255  165    0    0  255  165    0    0  102  102  102  255  510  420  178  255], MeshOffColor=[255  165    0    0  255  165    0    0  102  102  102  255    0    0    0  255], TimeStep=1/100}
      mask prompts: UniqueID "Parent Unique Identifier"; LightName "Light"; PivotName "Pivot"; TextureResources "Texture Resources"; ColorsObjectName "Light Fixture Color Object"; MeshOnColor "Light Fixture On Color"; MeshOffColor "Light Fixture Off Color"; TimeStep "Simulink time step"
      mask help:
      | The VisuActiveLight block provides a way for detailed animation of Light Sources, such as the indicator, brake, fog and main lights of a vehicle, or a light post.
      |
      | For more information, please click Help.
      mask init:
      | [tabledata] = mbxruntime.parameters.table(UniqueID,LightName,PivotName,TextureResources,ColorsObjectName,MeshOnColor,MeshOffColor);
      mask Help: eval('openHelp(209)')
      mask Display: image(imread('HeadLight.png'))
  wires:
  Honda_Pan_European_1_Indicator_front_right/1 -> Actuator/1

== system ACC_Scenario_006_cs/Honda_Pan_European_1_Indicator_rear_left ==
  Honda_Pan_European_1_Indicator_rear_left : Inport  Tag=inport/IndicatorRL  OutDataTypeStr=Bus: PRESCAN_VISULIGHTACTUATOR_DATA  SampleTime=1/100  BusOutputAsStruct=on
  Actuator : S-Function  FunctionName=sfun_VisuLightActuator  Parameters=mbxruntime.parameters.convert(UniqueID), mbxruntime.parameters.convert(LightName), mbxruntime.parameters.convert(PivotName), mbxruntime.parameters.convert(TextureResources), mbxruntime.parameters.convert(ColorsObjectName), mbxruntime.parameters.convert(MeshOnColor), mbxruntime.parameters.convert(MeshOffColor),tabledata, TimeStep  EnableBusSupport=off  mask(PreScan Sink Block: VisuActiveLight){UniqueID=356, LightName=Honda_Pan_European_1.LightActuator_3_IndicatorRL_ActiveLight, PivotName=Honda_Pan_European_1.IndicatorRL_pivot, TextureResources={ '21' 'LightMap\GeneralLight.png'}, ColorsObjectName=Honda_Pan_European_1.IndicatorRL, MeshOnColor=[255  165    0    0  255  165    0    0  102  102  102  255  510  420  178  255], MeshOffColor=[255  165    0    0  255  165    0    0  102  102  102  255    0    0    0  255], TimeStep=1/100}
      mask prompts: UniqueID "Parent Unique Identifier"; LightName "Light"; PivotName "Pivot"; TextureResources "Texture Resources"; ColorsObjectName "Light Fixture Color Object"; MeshOnColor "Light Fixture On Color"; MeshOffColor "Light Fixture Off Color"; TimeStep "Simulink time step"
      mask help:
      | The VisuActiveLight block provides a way for detailed animation of Light Sources, such as the indicator, brake, fog and main lights of a vehicle, or a light post.
      |
      | For more information, please click Help.
      mask init:
      | [tabledata] = mbxruntime.parameters.table(UniqueID,LightName,PivotName,TextureResources,ColorsObjectName,MeshOnColor,MeshOffColor);
      mask Help: eval('openHelp(209)')
      mask Display: image(imread('HeadLight.png'))
  wires:
  Honda_Pan_European_1_Indicator_rear_left/1 -> Actuator/1

== system ACC_Scenario_006_cs/Honda_Pan_European_1_Indicator_rear_right ==
  Honda_Pan_European_1_Indicator_rear_right : Inport  Tag=inport/IndicatorRR  OutDataTypeStr=Bus: PRESCAN_VISULIGHTACTUATOR_DATA  SampleTime=1/100  BusOutputAsStruct=on
  Actuator : S-Function  FunctionName=sfun_VisuLightActuator  Parameters=mbxruntime.parameters.convert(UniqueID), mbxruntime.parameters.convert(LightName), mbxruntime.parameters.convert(PivotName), mbxruntime.parameters.convert(TextureResources), mbxruntime.parameters.convert(ColorsObjectName), mbxruntime.parameters.convert(MeshOnColor), mbxruntime.parameters.convert(MeshOffColor),tabledata, TimeStep  EnableBusSupport=off  mask(PreScan Sink Block: VisuActiveLight){UniqueID=356, LightName=Honda_Pan_European_1.LightActuator_4_IndicatorRR_ActiveLight, PivotName=Honda_Pan_European_1.IndicatorRR_pivot, TextureResources={ '21' 'LightMap\GeneralLight.png'}, ColorsObjectName=Honda_Pan_European_1.IndicatorRR, MeshOnColor=[255  165    0    0  255  165    0    0  102  102  102  255  510  420  178  255], MeshOffColor=[255  165    0    0  255  165    0    0  102  102  102  255    0    0    0  255], TimeStep=1/100}
      mask prompts: UniqueID "Parent Unique Identifier"; LightName "Light"; PivotName "Pivot"; TextureResources "Texture Resources"; ColorsObjectName "Light Fixture Color Object"; MeshOnColor "Light Fixture On Color"; MeshOffColor "Light Fixture Off Color"; TimeStep "Simulink time step"
      mask help:
      | The VisuActiveLight block provides a way for detailed animation of Light Sources, such as the indicator, brake, fog and main lights of a vehicle, or a light post.
      |
      | For more information, please click Help.
      mask init:
      | [tabledata] = mbxruntime.parameters.table(UniqueID,LightName,PivotName,TextureResources,ColorsObjectName,MeshOnColor,MeshOffColor);
      mask Help: eval('openHelp(209)')
      mask Display: image(imread('HeadLight.png'))
  wires:
  Honda_Pan_European_1_Indicator_rear_right/1 -> Actuator/1
